simulink model "Estimador_DB_Caso_1"  (R2023a)
settings: Solver=VariableStepAuto  StartTime=0.0  StopTime=7  MaxStep=0.001  MinStep=0.0001  RelTol=1e-3  EnableMultiTasking=on
undefined symbols (not defined in the file): A, B, Cn, g, g0, K, Ke, l, M, m
settings Model: Creator=54115  LastModifiedBy=franc
settings SolverCC: AlgebraicLoopSolver=TrustRegion
settings DataIOCC: ReturnWorkspaceOutputs=off
settings OptimizationCC: LifeSpan=inf
settings DebuggingCC: UnconnectedInputMsg=warning  UnconnectedOutputMsg=warning  UnconnectedLineMsg=warning  SFUnexpectedBacktrackingDiag=warning  SFNoUnconditionalDefaultTransitionDiag=warning  ArithmeticOperatorsInVariantConditions=warning
settings ModelReferenceCC: EnableRefExpFcnMdlSchedulingChecks=on
settings SFSimCC: SimUseLocalCustomCode=off  CustomCodeUndefinedFunction=UseInterfaceOnly
settings RTWCC: RTWUseLocalCustomCode=off
settings CodeAppCC: StateflowObjectComments=on
settings GRTTargetCC: TargetLangStandard=C89/C90 (ANSI)
settings ConfigComp: CovMetricSettings=dw  CovSaveCumulativeToWorkspaceVar=on  CovSaveSingleToWorkspaceVar=on  CovExternalEMLEnable=off

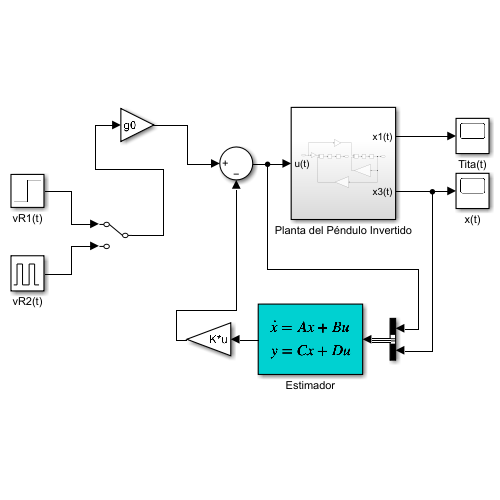
[thumbnail: Simulink's stored preview of the top-level diagram]
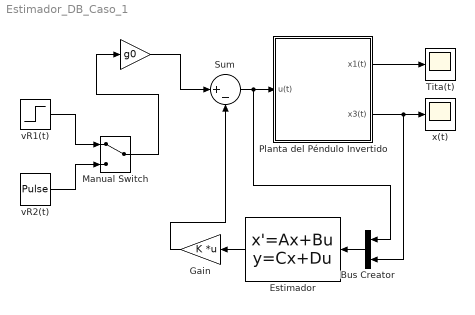
== system Estimador_DB_Caso_1 ==
  " " : Gain  Gain=g0
  Bus Creator : BusCreator  Inputs=2
  Estimador : StateSpace  A=A-Ke*Cn  B=[B Ke]  C=eye(4)  D=[0 0 0 0;0 0 0 0]'  InitialCondition=0
  Gain : Gain  Gain=K  Multiplication=Matrix(K*u)
  Manual Switch : ManualSwitch
  Planta del Péndulo Invertido : Subsystem
  Sum : Sum  Inputs=|+-
  Tita(t) : Scope
  vR1(t) : Step  Time=0  SampleTime=0
  vR2(t) : DiscretePulseGenerator  PulseType=Time based  PulseWidth=5
  x(t) : Scope
  wires:
  Estimador/1 -> Gain/1
  Sum/1 -> Planta del Péndulo Invertido/1(u(t)), Bus Creator/1
  Bus Creator/1 -> Estimador/1
  Gain/1 -> Sum/2
  " "/1 -> Sum/1
  Planta del Péndulo Invertido/1(x1(t)) -> Tita(t)/1
  Planta del Péndulo Invertido/2(x3(t)) -> x(t)/1, Bus Creator/2
  Manual Switch/1 -> " "/1
  vR1(t)/1 -> Manual Switch/1
  vR2(t)/1 -> Manual Switch/2

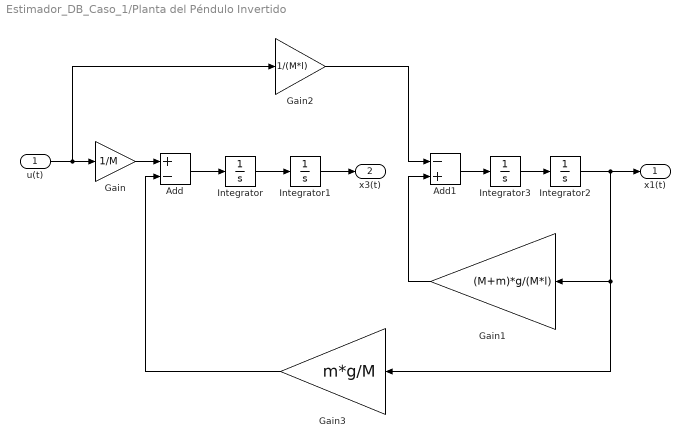
== system Estimador_DB_Caso_1/Planta del Péndulo Invertido ==
  u(t) : Inport
  Add : Sum  Inputs=+-
  Add1 : Sum  Inputs=-+
  Gain : Gain  Gain=1/M
  Gain1 : Gain  Gain=(M+m)*g/(M*l)
  Gain2 : Gain  Gain=1/(M*l)
  Gain3 : Gain  Gain=m*g/M
  Integrator{,1..3} (4 alike) : Integrator
  x1(t) : Outport
  x3(t) : Outport  Port=2
  wires:
  Add1/1 -> Integrator3/1
  Gain1/1 -> Add1/2
  Gain/1 -> Add/1
  Integrator/1 -> Integrator1/1
  Integrator1/1 -> x3(t)/1
  Gain2/1 -> Add1/1
  Gain3/1 -> Add/2
  Integrator3/1 -> Integrator2/1
  Integrator2/1 -> x1(t)/1, Gain3/1, Gain1/1
  u(t)/1 -> Gain2/1, Gain/1
  Add/1 -> Integrator/1
